simulink model "do_OFDM0_sim"  (Simulink 6.6)
settings: Solver=ode45  StartTime=0.0  StopTime=10.0  RelTol=1e-3
values from neighbouring files (symbols this model uses):
  b = 2    [e1.m]
  Nfft = 128    [e1.m]
  Ng = 16    [e1.m]
  Nsym = Nfft+Ng    (= 144)    [e1.m]
  SNRbdB = 10    [e1.m]
undefined symbols (not defined in the file or in its folder): get, magnitude, Nframe
libraries: simulink x3, dspstat3 x3, commsink2 x2, dspxfrm3 x2, dspindex x2, commdigbbndam3 x2, dspsnks4 x2, commchan3 x1, commrandsrc2 x1, dspobslib x1
settings Model: Creator=Won Y. Yang  LastModifiedBy=Wyyang

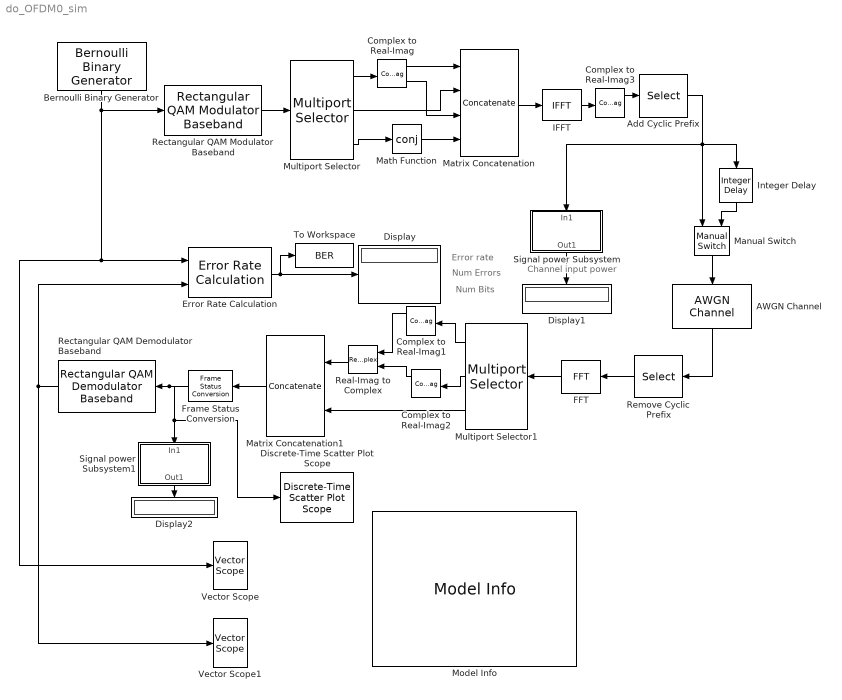
== system do_OFDM0_sim ==
  note: Error rate
  note: Num Errors
  note: Num Bits
  note: Channel input power
  AWGN Channel : commchan3/AWGN Channel  Orientation=down  SystemSampleTime=-1  seed=67  noiseMode="Signal to noise ratio  (Eb/No)"  EbNodB=SNRbdB-3  EsNodB=SNRbdB-3+10*log10(Nframe)  SNRdB=SNRbdB+10*log10(b)  bitsPerSym=Nblock  Ps=1/Nfft  Tsym=Tsym  variance=1
  Add Cyclic Prefix : Selector  IndexOptions=Index vector (dialog)  Indices=[Nfft-Ng+1:Nfft 1:Nfft]  OutputSizes=1  InputPortWidth=Nfft
  Bernoulli Binary Generator : commrandsrc2/Bernoulli Binary Generator  Orientation=down  DialogController=commDDGCreate  DialogControllerArgs=DataTag0  SystemSampleTime=-1  P=0.5  seed=61  Ts=Tsym/Nblock  frameBased=on  sampPerFrame=Nblock  orient=off  outDataType=double
  Complex to Real-Imag : ComplexToRealImag
  Complex to Real-Imag1 : ComplexToRealImag  Orientation=left
  Complex to Real-Imag2 : ComplexToRealImag  Orientation=left
  Complex to Real-Imag3 : ComplexToRealImag
  Discrete-Time Scatter Plot Scope : commsink2/Discrete-Time Scatter Plot Scope  Tag=ScatterPlot  SystemSampleTime=-1  sampPerSymb=1  offsetEye=0  numTraces=100  numNewFrames=100  LineMarkers=.  LineColors=b  fading=off  render=on  AxisGrid=on  xMin=-3.3  xMax=3.315  yMin=-3.3  yMax=3.315  inphaseLabel=In-phase Amplitude  quadratureLabel=Quadrature Amplitude  openScopeAtSimStart=on  FrameNumber=off  FigPos=get(0,'defaultfigureposition');  figTitle=Scatter Plot  numLinesMax=8  block_type_=scatter
  Display : Display
  Display1 : Display
      settings: Orientation=down
  Display2 : Display
      settings: Orientation=down
  Error Rate Calculation : commsink2/Error Rate Calculation  N=0  st_delay=0  cp_mode=Entire frame  subframe=[]  PMode=Port  WsName=ErrorVec  RsMode2=off  stop=off  numErr=100  maxBits=4e6
  FFT : dspxfrm3/FFT  Orientation=left  DialogController=dspDDGCreate  DialogControllerArgs=DataTag1  CompMethod=Table lookup  TableOpt=Speed  BitRevOrder=off  InheritFFTLength=on  FFTLength=64  SkipNorm=on  roundingMode=Floor  overflowMode=off
  Frame Status Conversion : dspobslib/Frame Status Conversion  Orientation=left  SystemSampleTime=-1  growRefPort=off  outframe=Frame-based
  IFFT : dspxfrm3/IFFT  DialogController=dspDDGCreate  DialogControllerArgs=DataTag2  CompMethod=Table lookup  TableOpt=Speed  BitRevOrder=off  cs_in=off  SkipNorm=off  InheritFFTLength=on  FFTLength=64  mode=Complex  roundingMode=Floor  overflowMode=off
  Integer Delay : simulink/Discrete/Integer Delay  Orientation=down  vinit=0.0  samptime=-1  NumDelays=1
  Manual Switch : simulink/Signal Routing/Manual Switch  Orientation=down  SystemSampleTime=-1  sw=1  action=0  varsize=off
  Math Function : Math  Operator=conj  SaturateOnIntegerOverflow=on
  Matrix Concatenation : Concatenate  NumInputs=4  Mode=Multidimensional array
  Matrix Concatenation1 : Concatenate  Orientation=left  Mode=Multidimensional array
  Model Info : simulink/Model-Wide Utilities/Model Info  SystemSampleTime=-1  InitialBlockCM=None  BlockCM=None  Frame=on  DisplayStringWithTags=|  HorizontalTextAlignment=Left  LeftAlignmentValue=0.02  SourceBlockDiagram=do_OFDM0_sim  TagMaxNumber=20
      | b=4; M=2^b; 
      | Nfft=128; Nffth=Nfft/2; 
      | Nblock=Nffth*b;
      | Ng=16; % Length of Guard interval or CP 
      | Nsym=Nfft+Ng; Tsym=0.001;
      | g=[0 1 0 0]; lc=length(g); 
      | [gmax,d1]=max(g); d=d1-1; 
      | lx=2*Nsym; lr=lx+Nsym; 
      | SNRbdB=10; 
      | SNRb=10^(SNRbdB/10); 
      | sigma=sqrt(1/(SNRb*Nblock))
      | prob_error(SNRbdB,'QAM',b,'BER')
  Multiport Selector : dspindex/Multiport Selector  rowsOrCols=Rows  idxCellArray={1,2:Nffth,Nffth:-1:2}  idxErrMode=Clip Index
  Multiport Selector1 : dspindex/Multiport Selector  Orientation=left  rowsOrCols=Rows  idxCellArray={1,Nffth+1,2:Nffth}  idxErrMode=Clip Index
  Real-Imag to Complex : RealImagToComplex  Orientation=left
  Rectangular QAM Demodulator Baseband : commdigbbndam3/Rectangular QAM Demodulator Baseband  Orientation=left  DialogController=commDDGCreate  DialogControllerArgs=DataTag3  M=M  PowType=Average Power  MinDist=2  AvgPow=1  PeakPow=1  Ph=0  Dec=Gray  Mapping=[0:15]  OutType=Bit  DecType=Hard decision  VarSource=Dialog  Variance=1  outDtype1=Inherit via internal rule  outDtype2=Inherit via internal rule  derotateFactorWordLen=16  denormFactorWordLen=16  prodOutWordLen=32  prodOutRoundingMode=Floor  prodOutOverflowMode=Wrap  sumWordLen=32
  Rectangular QAM Modulator Baseband : commdigbbndam3/Rectangular QAM Modulator Baseband  M=M  InType=Bit  Enc=Gray  Mapping=[0:15]  PowType=Average Power  MinDist=b  AvgPow=1  PeakPow=1  Ph=0  outDtype=double  outWordLen=16  outUDDataType=sfix(16)  outFracLenMode=Best precision  outFracLen=15
  Remove Cyclic Prefix : Selector  Orientation=left  IndexOptions=Index vector (dialog)  Indices=[Ng+1:Nsym]  OutputSizes=1  InputPortWidth=Nsym
  Signal power Subsystem : Subsystem  Orientation=down
  Signal power Subsystem1 : Subsystem  Orientation=down
  To Workspace : ToWorkspace  VariableName=BER  SampleTime=-1  SaveFormat=Array
      settings: MaxDataPoints=1
  Vector Scope : dspsnks4/Vector Scope  DialogController=dspdialog.VectorScope  DialogControllerArgs=DataTag7  ScopeProperties=on  Domain=Time  HorizSpan=2  DisplayProperties=off  AxisGrid=on  Memory=off  FrameNumber=on  AxisLegend=off  AxisZoom=off  OpenScopeAtSimStart=on  OpenScopeImmediately=off  FigPos=get(0,'defaultfigureposition')  AxisProperties=off  XUnits=Hertz  XRange=[0...Fs/2]  InheritXIncr=on  XIncr=1  XLabel=Time  XLimit=Auto  XMin=0  XMax=1  XStart=0  YUnits=dB  YLabel=Amplitude  LineProperties=off
      settings: YMin=-10  YMax=10
  Vector Scope1 : dspsnks4/Vector Scope  DialogController=dspdialog.VectorScope  DialogControllerArgs=DataTag8  ScopeProperties=on  Domain=Time  HorizSpan=2  DisplayProperties=off  AxisGrid=on  Memory=off  FrameNumber=on  AxisLegend=off  AxisZoom=off  OpenScopeAtSimStart=on  OpenScopeImmediately=off  FigPos=get(0,'defaultfigureposition')  AxisProperties=off  XUnits=Hertz  XRange=[0...Fs/2]  InheritXIncr=on  XIncr=1  XLabel=Time  XLimit=Auto  XMin=0  XMax=1  XStart=0  YUnits=dB  YLabel=Amplitude  LineProperties=off
      settings: YMin=-10  YMax=10
  wires:
  Bernoulli Binary Generator/1 -> Rectangular QAM Modulator Baseband/1, Error Rate Calculation/1, Vector Scope/1
  Add Cyclic Prefix/1 -> Signal power Subsystem/1(In1), Integer Delay/1, Manual Switch/1
  Rectangular QAM Modulator Baseband/1 -> Multiport Selector/1
  Multiport Selector/1 -> Complex to Real-Imag/1
  Complex to Real-Imag/1 -> Matrix Concatenation/1
  Complex to Real-Imag/2 -> Matrix Concatenation/3
  Multiport Selector/2 -> Matrix Concatenation/2
  Multiport Selector/3 -> Math Function/1
  Math Function/1 -> Matrix Concatenation/4
  Matrix Concatenation/1 -> IFFT/1
  AWGN Channel/1 -> Remove Cyclic Prefix/1
  Remove Cyclic Prefix/1 -> FFT/1
  FFT/1 -> Multiport Selector1/1
  Rectangular QAM Demodulator Baseband/1 -> Error Rate Calculation/2, Vector Scope1/1
  Error Rate Calculation/1 -> Display/1, To Workspace/1
  Real-Imag to Complex/1 -> Matrix Concatenation1/1
  Multiport Selector1/3 -> Matrix Concatenation1/2
  Matrix Concatenation1/1 -> Frame Status Conversion/1
  Frame Status Conversion/1 -> Rectangular QAM Demodulator Baseband/1, Signal power Subsystem1/1(In1), Discrete-Time Scatter Plot Scope/1
  Multiport Selector1/2 -> Complex to Real-Imag2/1
  Multiport Selector1/1 -> Complex to Real-Imag1/1
  Complex to Real-Imag1/1 -> Real-Imag to Complex/1
  Complex to Real-Imag2/1 -> Real-Imag to Complex/2
  Signal power Subsystem/1(Out1) -> Display1/1
  IFFT/1 -> Complex to Real-Imag3/1
  Complex to Real-Imag3/1 -> Add Cyclic Prefix/1
  Signal power Subsystem1/1(Out1) -> Display2/1
  Manual Switch/1 -> AWGN Channel/1
  Integer Delay/1 -> Manual Switch/2

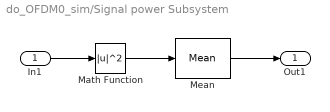
== system do_OFDM0_sim/Signal power Subsystem ==
  In1 : Inport
  Math Function : Math  Operator=magnitude^2  SaturateOnIntegerOverflow=on
  Mean : dspstat3/Mean  DialogController=dspDDGCreate  DialogControllerArgs=DataTag4  run=on  reset_popup=None  roundingMode=Floor  overflowMode=off
  Out1 : Outport
  wires:
  Mean/1 -> Out1/1
  In1/1 -> Math Function/1
  Math Function/1 -> Mean/1

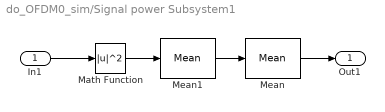
== system do_OFDM0_sim/Signal power Subsystem1 ==
  In1 : Inport
  Math Function : Math  Operator=magnitude^2  SaturateOnIntegerOverflow=on
  Mean : dspstat3/Mean  DialogController=dspDDGCreate  DialogControllerArgs=DataTag5  run=on  reset_popup=None  roundingMode=Floor  overflowMode=off
  Mean1 : dspstat3/Mean  DialogController=dspDDGCreate  DialogControllerArgs=DataTag6  run=off  reset_popup=None  roundingMode=Floor  overflowMode=off
  Out1 : Outport
  wires:
  Mean/1 -> Out1/1
  In1/1 -> Math Function/1
  Math Function/1 -> Mean1/1
  Mean1/1 -> Mean/1
